simulink model "DynamicPhysicalModel"  (R2025a)
settings: Solver=FixedStepAuto  StartTime=0.0  StopTime=10.0  RelTol=1e-3
undefined symbols (not defined in the file): c, J, L, M, R
settings Model: DataDictionary=Constants.sldd  Creator=levirogalla  LastModifiedBy=levirogalla

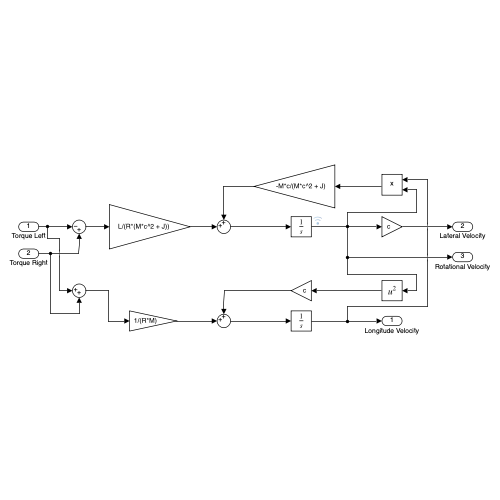
[thumbnail: Simulink's stored preview of the top-level diagram]
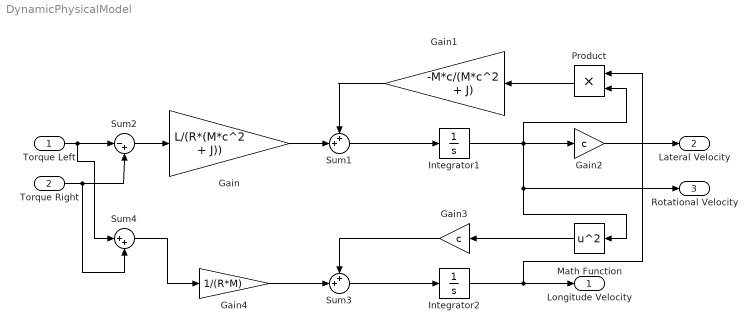
== system DynamicPhysicalModel ==
  Torque Left : Inport
  Torque Right : Inport  Port=2
  Gain : Gain  Gain=L/(R*(M*c^2 + J))
  Gain1 : Gain  Gain=-M*c/(M*c^2 + J)
  Gain2 : Gain  Gain=c
  Gain3 : Gain  Gain=c
  Gain4 : Gain  Gain=1/(R*M)
  Integrator1 : Integrator
  Integrator2 : Integrator
  Math Function : Math  Operator=square
  Product : Product
  Sum1 : Sum  Inputs=++|
  Sum2 : Sum  Inputs=|-+
  Sum3 : Sum  Inputs=++|
  Sum4 : Sum  Inputs=|++
  Longitude Velocity : Outport
  Lateral Velocity : Outport  Port=2
  Rotational Velocity : Outport  Port=3
  wires:
  Integrator1/1 -> Rotational Velocity/1, Math Function/1, Gain2/1, Product/2
  Math Function/1 -> Gain3/1
  Product/1 -> Gain1/1
  Gain3/1 -> Sum3/1
  Gain1/1 -> Sum1/1
  Sum3/1 -> Integrator2/1
  Sum1/1 -> Integrator1/1
  Torque Left/1 -> Sum4/1, Sum2/1
  Gain/1 -> Sum1/2
  Gain2/1 -> Lateral Velocity/1
  Integrator2/1 -> Longitude Velocity/1, Product/1
  Gain4/1 -> Sum3/2
  Sum2/1 -> Gain/1
  Torque Right/1 -> Sum4/2, Sum2/2
  Sum4/1 -> Gain4/1
